simulink model "Control_Model_Simulink"  (R2021a)
settings: Solver=VariableStepAuto  StartTime=0.0  StopTime=300  RelTol=1e-3
values from neighbouring files (symbols this model uses):
  Br = 2    [Matlab_Linear_Model.m]    (also in Matlab__Linear_Model.m = 20; Matlab__Linear_Model_2.m; Matlab__NonLinear_Model.m = 0.5; Mc1.mat)
  g = 9.81    [Fixed_Model.m]    (also in Matlab_Linear_Model.m; Matlab__Linear_Model.m; Matlab__Linear_Model_2.m; Matlab__NonLinear_Model.m)
  H = hip * cos(-beta)    [Matlab__Linear_Model.m]    (also in Matlab__NonLinear_Model.m = (hip * cos(-beta)))
  I = I1 + I2    (= 1.59448333333)    [Fixed_Model.m]    (also in Matlab_Linear_Model.m = 0.63768; Matlab__Linear_Model.m = 0.8924; Matlab__Linear_Model_2.m = 0.8924; Matlab__NonLinear_Model.m = 0.556904166667)
  l2x = (l1 + l2)/2 + l3x    (= 0.875)    [Fixed_Model.m]    (also in Matlab__Linear_Model.m = 0.65; Matlab__NonLinear_Model.m = 0.575)
  l3f = l3o + 0.15    (= 0.3)    [Matlab_Linear_Model.m]    (also in Matlab__Linear_Model.m; Matlab__Linear_Model_2.m; Matlab__NonLinear_Model.m; Mc1.mat)
  l3o = 0.3    [Fixed_Model.m]    (also in Matlab_Linear_Model.m = 0.15; Matlab__Linear_Model.m = 0.15; Matlab__Linear_Model_2.m = 0.15; Matlab__NonLinear_Model.m = 0.15)
  m2 = 2    [Fixed_Model.m]    (also in Matlab_Linear_Model.m = 1.4; Matlab__Linear_Model.m; Matlab__Linear_Model_2.m; Matlab__NonLinear_Model.m = 1.5)
  M2 = (F2*l2x)    (= -12.753)    [Matlab__Linear_Model.m]    (also in Matlab__NonLinear_Model.m = (F2*l2x*cos(theta)))
libraries: simulink x1
settings Model: Creator=DANI-TUF  LastModifiedBy=DANI-TUF

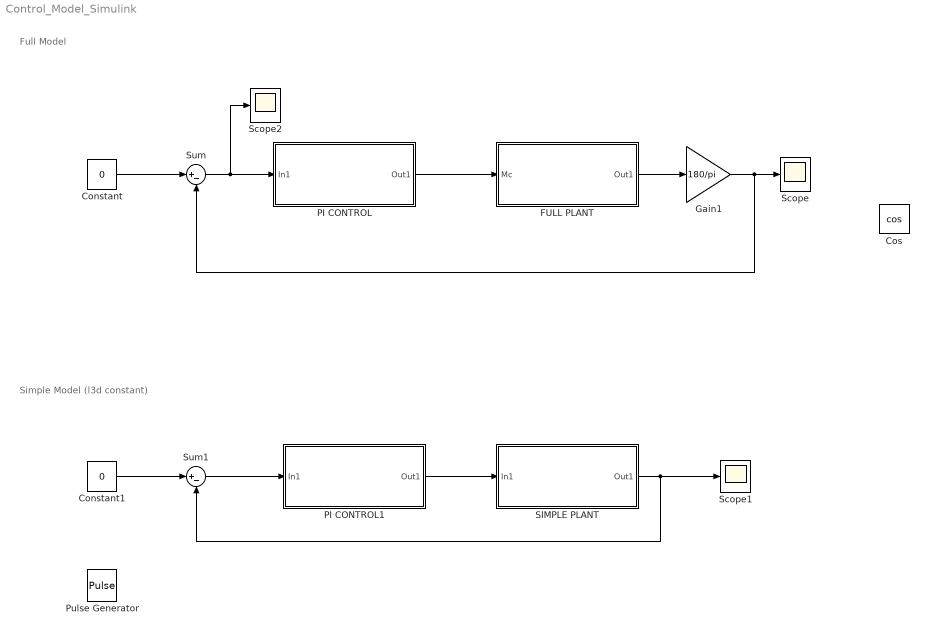
== system Control_Model_Simulink ==
  note: Simple Model (l3d constant)
  note: Full Model
  Constant : Constant  Value=0
  Constant1 : Constant  Value=0
  Cos : Trigonometry  Operator=cos
  FULL PLANT : Subsystem
  Gain1 : Gain  Gain=180/pi
  PI CONTROL : Subsystem
  PI CONTROL1 : Subsystem
  Pulse Generator : DiscretePulseGenerator  PulseType=Time based  Amplitude=10  Period=10  PulseWidth=10
  SIMPLE PLANT : Subsystem
  Scope : Scope
  Scope1 : Scope
  Scope2 : Scope
  Sum : Sum  Inputs=|+-
  Sum1 : Sum  Inputs=|+-
  wires:
  Constant1/1 -> Sum1/1
  SIMPLE PLANT/1(Out1) -> Scope1/1, Sum1/2
  PI CONTROL/1(Out1) -> FULL PLANT/1(Mc)
  Sum/1 -> Scope2/1, PI CONTROL/1(In1)
  Constant/1 -> Sum/1
  FULL PLANT/1(Out1) -> Gain1/1
  Sum1/1 -> PI CONTROL1/1(In1)
  PI CONTROL1/1(Out1) -> SIMPLE PLANT/1(In1)
  Gain1/1 -> Sum/2, Scope/1

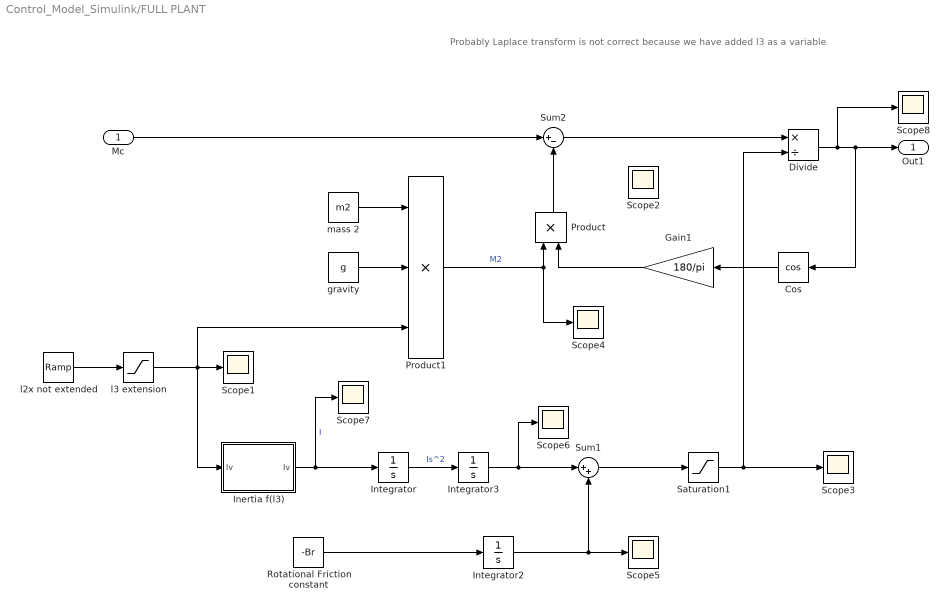
== system Control_Model_Simulink/FULL PLANT ==
  note: Probably Laplace transform is not correct because we have added l3 as a variable
  Mc : Inport
  Cos : Trigonometry  Operator=cos
  Divide : Product  Inputs=*/
  Gain1 : Gain  Gain=180/pi
  Inertia f(l3) : MATLAB Function  TreatAsAtomicUnit=on
  Integrator : Integrator
  Integrator2 : Integrator  LimitOutput=on  UpperSaturationLimit=2
  Integrator3 : Integrator  LimitOutput=on  UpperSaturationLimit=10e6  LowerSaturationLimit=0
  Product : Product
  Product1 : Product  Inputs=3
  Rotational Friction constant : Constant  Value=-Br
  Saturation1 : Saturate  UpperLimit=inf  LowerLimit=0.00001
  Scope{1..8} (8 alike) : Scope
  Sum1 : Sum  Inputs=|++
  Sum2 : Sum  Inputs=|+-
  gravity : Constant  Value=g
  l2x not extended : simulink/Sources/Ramp  slope=0.05  start=60  InitialOutput=l2x - l3f + l3o
  l3 extension : Saturate  UpperLimit=l2x  LowerLimit=l2x - l3f + l3o
  mass 2 : Constant  Value=m2
  Out1 : Outport
  wires:
  mass 2/1 -> Product1/1
  gravity/1 -> Product1/2
  l2x not extended/1 -> l3 extension/1
  l3 extension/1 -> Product1/3, Scope1/1, Inertia f(l3)/1(lv)
  Product1/1 -> Product/1, Scope4/1  "M2"
  Inertia f(l3)/1(Iv) -> Integrator/1, Scope7/1  "I"
  Integrator/1 -> Integrator3/1  "Is^2"
  Rotational Friction constant/1 -> Integrator2/1
  Sum1/1 -> Saturation1/1
  Sum2/1 -> Divide/1
  Saturation1/1 -> Scope3/1, Divide/2
  Integrator2/1 -> Sum1/2, Scope5/1
  Gain1/1 -> Product/2
  Divide/1 -> Scope8/1, Cos/1, Out1/1
  Cos/1 -> Gain1/1
  Integrator3/1 -> Sum1/1, Scope6/1
  Product/1 -> Sum2/2
  Mc/1 -> Sum2/1

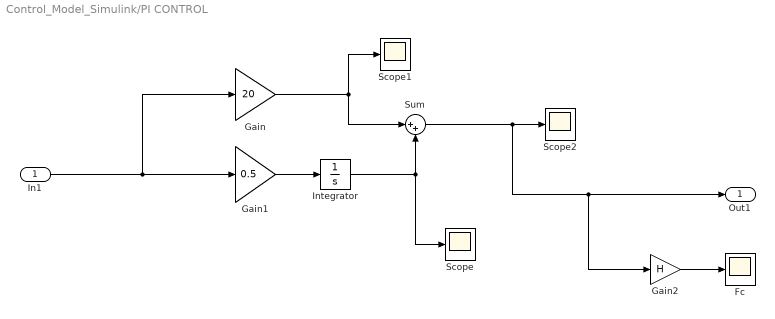
== system Control_Model_Simulink/PI CONTROL ==
  In1 : Inport
  Fc : Scope
  Gain : Gain  Gain=20
  Gain1 : Gain  Gain=0.5
  Gain2 : Gain  Gain=H
  Integrator : Integrator
  Scope : Scope
  Scope1 : Scope
  Scope2 : Scope
  Sum : Sum  Inputs=|++
  Out1 : Outport
  wires:
  Gain1/1 -> Integrator/1
  Integrator/1 -> Scope/1, Sum/2
  Gain/1 -> Sum/1, Scope1/1
  In1/1 -> Gain/1, Gain1/1
  Sum/1 -> Gain2/1, Out1/1, Scope2/1
  Gain2/1 -> Fc/1

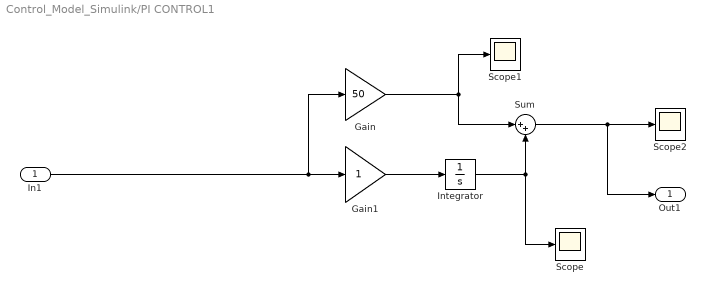
== system Control_Model_Simulink/PI CONTROL1 ==
  In1 : Inport
  Gain : Gain  Gain=50
  Gain1 : Gain
  Integrator : Integrator
  Scope : Scope
  Scope1 : Scope
  Scope2 : Scope
  Sum : Sum  Inputs=|++
  Out1 : Outport
  wires:
  Sum/1 -> Scope2/1, Out1/1
  Gain1/1 -> Integrator/1
  Integrator/1 -> Scope/1, Sum/2
  In1/1 -> Gain/1, Gain1/1
  Gain/1 -> Sum/1, Scope1/1

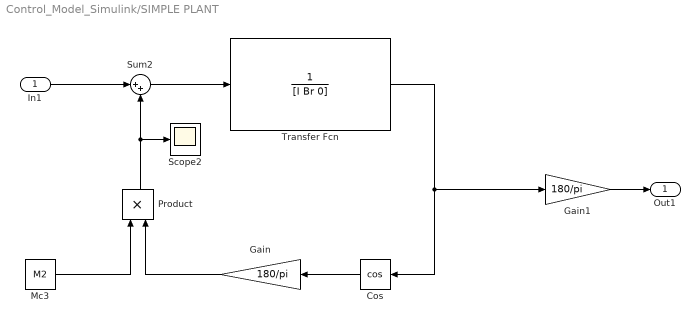
== system Control_Model_Simulink/SIMPLE PLANT ==
  In1 : Inport
  Cos : Trigonometry  Operator=cos
  Gain : Gain  Gain=180/pi
  Gain1 : Gain  Gain=180/pi
  Mc3 : Constant  Value=M2
  Product : Product
  Scope2 : Scope
  Sum2 : Sum  Inputs=|++
  Transfer Fcn : TransferFcn  Denominator=[I Br 0]
  Out1 : Outport
  wires:
  Cos/1 -> Gain/1
  Sum2/1 -> Transfer Fcn/1
  Gain/1 -> Product/2
  Mc3/1 -> Product/1
  Product/1 -> Scope2/1, Sum2/2
  In1/1 -> Sum2/1
  Gain1/1 -> Out1/1
  Transfer Fcn/1 -> Cos/1, Gain1/1

== matlab function Control_Model_Simulink/FULL PLANT/Inertia f(l3) ==
  data: lv input; Iv output
function Iv = fcn(lv)
% Box dimensions
t1 = 0.3; % height of box 1 (m)
l1 = 0.35; % lenght of box 1 (m)

t2 = 0.2; % height of box 2 (m)
l2 = 0.2; % lenght of box 2 (m)

% IT SHOULD BE ON f(x)
l3o = 0.3; % Initial linear actuator lenght (m)
m1 = 4.5;   % Mass of box 1 (big box) (kg)
m2 = 2.5;   % Mass of box 2 (little box) (kg)

len = l1/2 + l2/2 + l3o + lv;

I1 = (m1 * (t1^2 + l1^2))/12; % Rotational inertia of box 1 [Kg*m^2]
I2 = (m2 * (t2^2 + l2^2))/12 + (m2 * len^2);  % Rotational inertia of box 2 [Kg*m^2]

Iv = I1 + I2; % Rotational Inertia #CHECK
